simulink model "FOC_Test"  (R2022b)
settings: Solver=FixedStepDiscrete  StartTime=0.0  StopTime=10.0  FixedStep=0.0001  RelTol=1e-3
libraries: Rtunit12 x30, PowerElectronics x2, simulink x1, RtuBox x1
settings Model: Creator=LJ  LastModifiedBy=Administrator
settings SolverCC: AlgebraicLoopSolver=TrustRegion
settings DataIOCC: ReturnWorkspaceOutputs=off
settings OptimizationCC: ReuseModelBlockBuffer=on
settings DebuggingCC: UnderspecifiedInitializationDetection=Classic  MergeDetectMultiDrivingBlocksExec=none  UnconnectedInputMsg=warning  UnconnectedOutputMsg=warning  UnconnectedLineMsg=warning  ArithmeticOperatorsInVariantConditions=warning
settings ModelReferenceCC: EnableRefExpFcnMdlSchedulingChecks=on
settings SFSimCC: SimUseLocalCustomCode=off  CustomCodeUndefinedFunction=UseInterfaceOnly
settings RTWCC: RTWUseLocalCustomCode=off
settings CodeAppCC: StateflowObjectComments=on

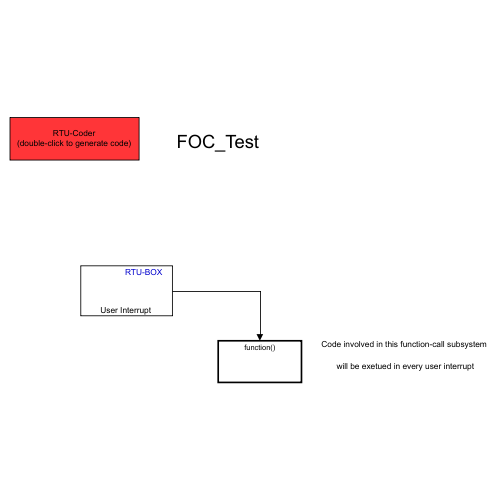
[thumbnail: Simulink's stored preview of the top-level diagram]
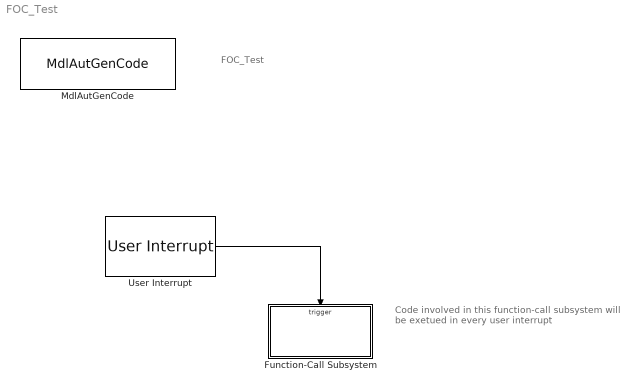
== system FOC_Test ==
  note: Code involved in this function-call subsystem
      |
      | will be exetued in every user interrupt
  note: FOC_Test
  Function-Call Subsystem : Subsystem  TreatAsAtomicUnit=on
  MdlAutGenCode : RtuBox/MdlAutGenCode
      settings: SourceProductName=RTU-BOX204 Toolbox
  User Interrupt : Rtunit12/User Interrupt  TimeEnable=User setting  TimeFreq=10
      settings: SourceProductName=RTU-BOX204 Toolbox
  wires:
  User Interrupt/1 -> Function-Call Subsystem/Trigger

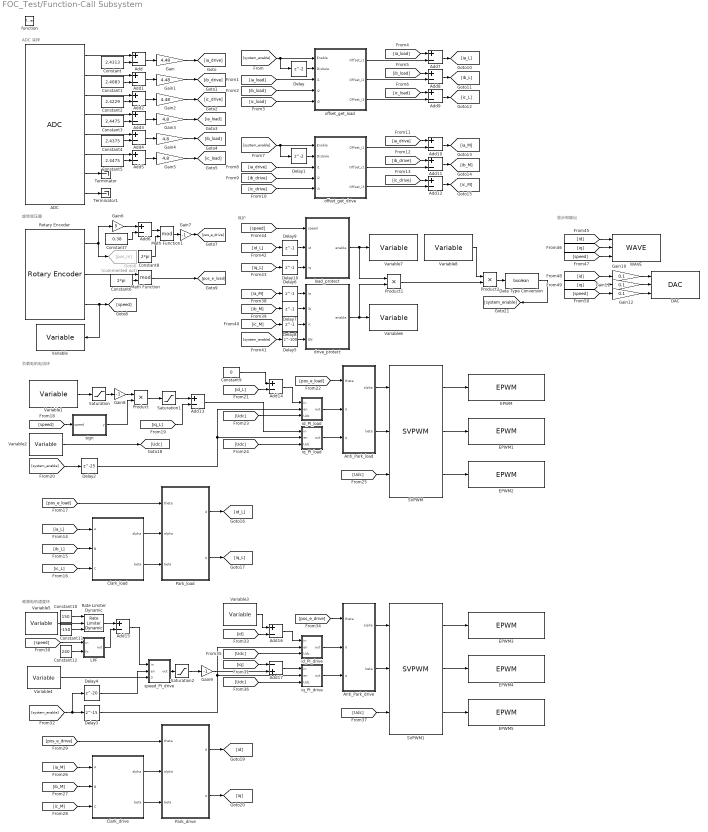
== system FOC_Test/Function-Call Subsystem ==
  note: 显示和输出
  note: 保护
  note: 负载电机电流环
  note: 旋转变压器
  note: ADC 采样
  note: 被测电机速度环
  function : TriggerPort  TriggerType=function-call  VariantControl=Variant
  " SVPWM" : PowerElectronics/ SVPWM
      settings: SourceProductName=RTU-BOX204 Toolbox
  " SVPWM1" : PowerElectronics/ SVPWM
      settings: SourceProductName=RTU-BOX204 Toolbox
  ADC : Rtunit12/ADC  SlotNo=ADC_A  InputSingleType=Single ended input and 16-bit resolution  numConversionsSingle=8  conv0=ADCIN00  GainEable1=on  Gain1=0.00030517578125  Offset1=0  conv1=ADCIN01  GainEable2=on  Gain2=0.00030517578125  Offset2=0  conv2=ADCIN02  GainEable3=on  Gain3=0.00030517578125  Offset3=0  conv3=ADCIN03  GainEable4=on  Gain4=0.00030517578125  Offset4=0  conv4=ADCIN04  GainEable5=on  Gain5=0.00030517578125  Offset5=0  conv5=ADCIN05  GainEable6=on  Gain6=0.00030517578125  Offset6=0  conv6=ADCIN06  GainEable7=on  Gain7=0.00030517578125  Offset7=0  conv7=ADCIN07  GainEable8=on  Gain8=0.00030517578125  Offset8=0  conv8=ADCIN01  GainEable9=off  Gain9=0.00015411376953125  Offset9=0  conv9=ADCIN01  GainEable10=off  Gain10=0.00015411376953125  Offset10=0  conv10=ADCIN01  GainEable11=off  Gain11=0.00015411376953125  Offset11=0  conv11=ADCIN01  GainEable12=off  Gain12=0.00015411376953125  Offset12=0  conv12=ADCIN01  GainEable13=off  Gain13=0.00015411376953125  Offset13=0  conv13=ADCIN01  GainEable14=off  Gain14=0.00015411376953125  Offset14=0  conv14=ADCIN01  GainEable15=off  Gain15=0.00015411376953125  Offset15=0  conv15=ADCIN01  GainEable16=off  Gain16=0.00015411376953125  Offset16=0  c28xmultiPort=on  AutoOffset=off
      settings: SourceProductName=RTU-BOX204 Toolbox
  Add{,1..16} (17 alike) : Sum  Inputs=+-  OutDataTypeStr=single  AccumDataTypeStr=single
  Add17 : Sum  Inputs=-+  OutDataTypeStr=single  AccumDataTypeStr=single
  Anti_Park_drive : MATLAB Function  TreatAsAtomicUnit=on
  Anti_Park_load : MATLAB Function  TreatAsAtomicUnit=on
  Clark_drive : MATLAB Function  TreatAsAtomicUnit=on
  Clark_load : MATLAB Function  TreatAsAtomicUnit=on
  Constant : Constant  Value=2.4313  OutDataTypeStr=single
  Constant1 : Constant  Value=2.4083  OutDataTypeStr=single
  Constant10 : Constant  Value=150  OutDataTypeStr=single
  Constant11 : Constant  Value=-150  OutDataTypeStr=single
  Constant12 : Constant  Value=240  OutDataTypeStr=single
  Constant2 : Constant  Value=2.4229  OutDataTypeStr=single
  Constant3 : Constant  Value=2.4475  OutDataTypeStr=single
  Constant4 : Constant  Value=2.4375  OutDataTypeStr=single
  Constant5 : Constant  Value=2.4475  OutDataTypeStr=single
  Constant6 : Constant  Value=2*pi  OutDataTypeStr=single
  Constant7 : Constant  Value=0.38  OutDataTypeStr=single
  Constant8 : Constant  Value=2*pi  OutDataTypeStr=single
  Constant9 : Constant  Value=0  OutDataTypeStr=single
  DAC : Rtunit12/DAC  useModule=A  Ts=-1  numConversionsSingle=3  conv0=DACOUTA0  conv1=DACOUTA1  conv2=DACOUTA2  conv3=DACOUTA0  conv4=DACOUTA0  conv5=DACOUTA0  conv6=DACOUTA0  conv7=DACOUTA0  conv8=DACOUT00  conv9=DACOUT00  conv10=DACOUT00  conv11=DACOUT00  conv12=DACOUT00  conv13=DACOUT00  conv14=DACOUT00  conv15=DACOUT00  dType=uint32  c28xmultiPort=on
      settings: SourceProductName=RTU-BOX204 Toolbox
  Data Type Conversion : DataTypeConversion  OutDataTypeStr=boolean  SaturateOnIntegerOverflow=off  RndMeth=Floor
  Delay : Delay  InitialCondition=0
  Delay1 : Delay  InitialCondition=0
  Delay{6..10} (5 alike) : Delay  DelayLength=1  InitialCondition=0
  Delay2 : Delay  DelayLength=25  InitialCondition=0
  Delay3 : Delay  DelayLength=15  InitialCondition=0
  Delay4 : Delay  DelayLength=20  InitialCondition=0
  Delay5 : Delay  DelayLength=100  InitialCondition=0
  EPWM : Rtunit12/EPWM  UserMode=Complimentary Signals Output  CHANNEL=4  EPWMA=EPWMA  LoadmodeA=CNT=0  LoadmodeB=CNT=0  STYLE=Triangle  DEADTIME=1  PhaseEnable=OFF  PhaseSlct=Dialog  PHASE=0  FreqSlct=Dialog  Frequency=10000  DutyUnit=Percentages  DutyInit=0.5  SynEnable=CTR=Zero  ChoppEnable=OFF  ChoppFrqDivd=5  ChoppCycFir=1  ChoppPulseCyc=1
      settings: SourceProductName=RTU-BOX204 Toolbox
  EPWM1 : Rtunit12/EPWM  UserMode=Complimentary Signals Output  CHANNEL=5  EPWMA=EPWMA  LoadmodeA=CNT=0  LoadmodeB=CNT=0  STYLE=Triangle  DEADTIME=1  PhaseEnable=ON  PhaseSlct=Dialog  PHASE=0  FreqSlct=Dialog  Frequency=10000  DutyUnit=Percentages  DutyInit=0.5  SynEnable=Synchronization Input  ChoppEnable=OFF  ChoppFrqDivd=5  ChoppCycFir=1  ChoppPulseCyc=1
      settings: SourceProductName=RTU-BOX204 Toolbox
  EPWM2 : Rtunit12/EPWM  UserMode=Complimentary Signals Output  CHANNEL=6  EPWMA=EPWMA  LoadmodeA=CNT=0  LoadmodeB=CNT=0  STYLE=Triangle  DEADTIME=1  PhaseEnable=ON  PhaseSlct=Dialog  PHASE=0  FreqSlct=Dialog  Frequency=10000  DutyUnit=Percentages  DutyInit=0.5  SynEnable=Synchronization Input  ChoppEnable=OFF  ChoppFrqDivd=5  ChoppCycFir=1  ChoppPulseCyc=1
      settings: SourceProductName=RTU-BOX204 Toolbox
  EPWM3 : Rtunit12/EPWM  UserMode=Complimentary Signals Output  CHANNEL=1  EPWMA=EPWMA  LoadmodeA=CNT=0  LoadmodeB=CNT=0  STYLE=Triangle  DEADTIME=1  PhaseEnable=OFF  PhaseSlct=Dialog  PHASE=0  FreqSlct=Dialog  Frequency=10000  DutyUnit=Percentages  DutyInit=0.5  SynEnable=CTR=Zero  ChoppEnable=OFF  ChoppFrqDivd=5  ChoppCycFir=1  ChoppPulseCyc=1
      settings: SourceProductName=RTU-BOX204 Toolbox
  EPWM4 : Rtunit12/EPWM  UserMode=Complimentary Signals Output  CHANNEL=2  EPWMA=EPWMA  LoadmodeA=CNT=0  LoadmodeB=CNT=0  STYLE=Triangle  DEADTIME=1  PhaseEnable=ON  PhaseSlct=Dialog  PHASE=0  FreqSlct=Dialog  Frequency=10000  DutyUnit=Percentages  DutyInit=0.5  SynEnable=Synchronization Input  ChoppEnable=OFF  ChoppFrqDivd=5  ChoppCycFir=1  ChoppPulseCyc=1
      settings: SourceProductName=RTU-BOX204 Toolbox
  EPWM5 : Rtunit12/EPWM  UserMode=Complimentary Signals Output  CHANNEL=3  EPWMA=EPWMA  LoadmodeA=CNT=0  LoadmodeB=CNT=0  STYLE=Triangle  DEADTIME=1  PhaseEnable=ON  PhaseSlct=Dialog  PHASE=0  FreqSlct=Dialog  Frequency=10000  DutyUnit=Percentages  DutyInit=0.5  SynEnable=Synchronization Input  ChoppEnable=OFF  ChoppFrqDivd=5  ChoppCycFir=1  ChoppPulseCyc=1
      settings: SourceProductName=RTU-BOX204 Toolbox
  Gain : Gain  Gain=4.48  ParamDataTypeStr=single  OutDataTypeStr=single
  Gain1 : Gain  Gain=4.48  ParamDataTypeStr=single  OutDataTypeStr=single
  Gain10 : Gain  Gain=0.1  ParamDataTypeStr=single  OutDataTypeStr=single
  Gain11 : Gain  Gain=0.1  ParamDataTypeStr=single  OutDataTypeStr=single
  Gain12 : Gain  Gain=0.1  ParamDataTypeStr=single  OutDataTypeStr=single
  Gain2 : Gain  Gain=4.48  ParamDataTypeStr=single  OutDataTypeStr=single
  Gain3 : Gain  Gain=4.8  ParamDataTypeStr=single  OutDataTypeStr=single
  Gain4 : Gain  Gain=4.8  ParamDataTypeStr=single  OutDataTypeStr=single
  Gain5 : Gain  Gain=4.8  ParamDataTypeStr=single  OutDataTypeStr=single
  Gain6 : Gain  Gain=5  ParamDataTypeStr=single  OutDataTypeStr=single
  Gain7 : Gain  Gain=-1  ParamDataTypeStr=single  OutDataTypeStr=single
  Gain8 : Gain  Gain=-1  ParamDataTypeStr=single  OutDataTypeStr=single
  Gain9 : Gain  Gain=-1  ParamDataTypeStr=single  OutDataTypeStr=single
  Goto6 : Goto  Commented=on  GotoTag=pos_m
  LPF : Subsystem
  Math Function : Math  Operator=mod
  Math Function1 : Math  Operator=mod
  Park_drive : MATLAB Function  TreatAsAtomicUnit=on
  Park_load : MATLAB Function  TreatAsAtomicUnit=on
  Product : Product  OutDataTypeStr=single
  Product1 : Product  OutDataTypeStr=single
  Product2 : Product  OutDataTypeStr=single
  Rate Limiter Dynamic : simulink/Discontinuities/Rate Limiter Dynamic
  Rotary Encoder : Rtunit12/Rotary Encoder  ChipSlct=0  Position_Compensate=0  Pole=4  Pole_Encoder=1  Bit_Encoder=16
      settings: SourceProductName=RTU-BOX204 Toolbox
  Saturation : Saturate  UpperLimit=1  LowerLimit=-1  OutDataTypeStr=single
  Saturation1 : Saturate  UpperLimit=2  LowerLimit=-2  OutDataTypeStr=single
  Saturation2 : Saturate  UpperLimit=3  LowerLimit=-3  OutDataTypeStr=single
  Terminator : Terminator
  Terminator1 : Terminator
  Variable : Rtunit12/Variable  nameStr=speed  DType=Single  Rw=Read only  InitVale=2  uint=rpm
      settings: SourceProductName=RTU-BOX204 Toolbox
  Variable1 : Rtunit12/Variable  nameStr=iq_load_ref  DType=Single  Rw=Read and Write  InitVale=0  uint=A
      settings: SourceProductName=RTU-BOX204 Toolbox
  Variable2 : Rtunit12/Variable  nameStr=Udc  DType=Single  Rw=Read and Write  InitVale=60  uint=V
      settings: SourceProductName=RTU-BOX204 Toolbox
  Variable3 : Rtunit12/Variable  nameStr=id_ref  DType=Single  Rw=Read and Write  InitVale=0  uint=A
      settings: SourceProductName=RTU-BOX204 Toolbox
  Variable4 : Rtunit12/Variable  nameStr=iq_limit  DType=Single  Rw=Read and Write  InitVale=3  uint=A
      settings: SourceProductName=RTU-BOX204 Toolbox
  Variable5 : Rtunit12/Variable  nameStr=speed_ref  DType=Single  Rw=Read and Write  InitVale=0  uint=rpm
      settings: SourceProductName=RTU-BOX204 Toolbox
  Variable6 : Rtunit12/Variable  nameStr=drive_motor_protect  DType=Single  Rw=Read only  InitVale=2
      settings: SourceProductName=RTU-BOX204 Toolbox
  Variable7 : Rtunit12/Variable  nameStr=load_motor_protect  DType=Single  Rw=Read only  InitVale=2
      settings: SourceProductName=RTU-BOX204 Toolbox
  Variable8 : Rtunit12/Variable  nameStr=system_enable  DType=Boolean  Rw=Read and Write  InitVale=0
      settings: SourceProductName=RTU-BOX204 Toolbox
  WAVE : Rtunit12/WAVE  RcvMode=Rtunit Studio  NumChnnl=3  Wave1Name=id  Wave1Max=4  Wave1Min=-4  Wave2Name=iq  Wave2Max=4  Wave2Min=-4  Wave3Name=speed  Wave3Max=600  Wave3Min=-600  Wave4Name=wave4  Wave4Max=10  Wave4Min=-10  Wave5Name=wave5  Wave5Max=10  Wave5Min=-10  Wave6Name=wave6  Wave6Max=10  Wave6Min=-10  Wave7Name=wave7  Wave7Max=10  Wave7Min=-10  Wave8Name=wave8  Wave8Max=10  Wave8Min=-10
      settings: SourceProductName=RTU-BOX204 Toolbox
  drive_protect : MATLAB Function  TreatAsAtomicUnit=on
  id_PI_drive : Subsystem
  id_PI_load : Subsystem
  iq_PI_drive : Subsystem
  iq_PI_load : Subsystem
  load_protect : MATLAB Function  TreatAsAtomicUnit=on
  offset_get_drive : MATLAB Function  TreatAsAtomicUnit=on
  offset_get_load : MATLAB Function  TreatAsAtomicUnit=on
  sign : MATLAB Function  TreatAsAtomicUnit=on
  speed_PI_drive : Subsystem
  wires:
  Constant/1 -> Add/2
  ADC/1 -> Add/1
  Add/1 -> Gain/1
  Gain/1 -> [ia_drive]
  Constant1/1 -> Add1/2
  Gain1/1 -> [ib_drive]
  ADC/2 -> Add1/1
  Add1/1 -> Gain1/1
  Add2/1 -> Gain2/1
  ADC/3 -> Add2/1
  Constant2/1 -> Add2/2
  Gain2/1 -> [ic_drive]
  Gain5/1 -> [ic_load]
  Constant5/1 -> Add5/2
  Constant3/1 -> Add3/2
  Add5/1 -> Gain5/1
  Gain3/1 -> [ia_load]
  Add4/1 -> Gain4/1
  ADC/5 -> Add4/1
  Constant4/1 -> Add4/2
  Gain4/1 -> [ib_load]
  ADC/6 -> Add5/1
  ADC/4 -> Add3/1
  Add3/1 -> Gain3/1
  ADC/7 -> Terminator/1
  ADC/8 -> Terminator1/1
  Rotary Encoder/1 -> Gain6/1, Goto6/1
  Rotary Encoder/2 -> Math Function/1
  Rotary Encoder/3 -> Variable/1, [speed]
  Constant6/1 -> Math Function/2
  Math Function/1 -> [pos_e_load]
  Gain6/1 -> Add6/1
  Constant7/1 -> Add6/2
  Add6/1 -> Math Function1/1
  Math Function1/1 -> Gain7/1
  Constant8/1 -> Math Function1/2
  Gain7/1 -> [pos_e_drive]
  [system_enable] -> Delay/1, offset_get_load/1(Enable)
  Delay/1 -> offset_get_load/2(Disbale)
  [ia_load] -> offset_get_load/3(i1)
  [ic_load] -> offset_get_load/5(i3)
  [ib_load] -> offset_get_load/4(i2)
  offset_get_load/1(Offset_i1) -> Add7/2
  [ia_load] -> Add7/1
  offset_get_load/2(Offset_i2) -> Add8/2
  [ib_load] -> Add8/1
  [ic_load] -> Add9/1
  offset_get_load/3(Offset_i3) -> Add9/2
  Add7/1 -> [ia_L]
  Add8/1 -> [ib_L]
  Add9/1 -> [ic_L]
  offset_get_drive/1(Offset_i1) -> Add10/2
  offset_get_drive/3(Offset_i3) -> Add12/2
  [ib_drive] -> Add11/1
  Add10/1 -> [ia_M]
  offset_get_drive/2(Offset_i2) -> Add11/2
  [ia_drive] -> Add10/1
  Add12/1 -> [ic_M]
  [system_enable] -> Delay1/1, offset_get_drive/1(Enable)
  [ic_drive] -> offset_get_drive/5(i3)
  Add11/1 -> [ib_M]
  [ia_drive] -> offset_get_drive/3(i1)
  Delay1/1 -> offset_get_drive/2(Disbale)
  [ib_drive] -> offset_get_drive/4(i2)
  [ic_drive] -> Add12/1
  [ia_L] -> Clark_load/1(A)
  [ib_L] -> Clark_load/2(B)
  [ic_L] -> Clark_load/3(C)
  Clark_load/1(alpha) -> Park_load/2(alpha)
  Clark_load/2(beta) -> Park_load/3(beta)
  [pos_e_load] -> Park_load/1(theta)
  Park_load/1(d) -> [id_L]
  Park_load/2(q) -> [iq_L]
  Variable1/1 -> Saturation/1
  Saturation/1 -> Gain8/1
  Gain8/1 -> Product/1
  sign/1(y) -> Product/2
  [speed] -> sign/1(speed)
  Product/1 -> Saturation1/1
  Saturation1/1 -> Add13/1
  [iq_L] -> Add13/2
  [system_enable] -> Delay2/1
  Delay2/1 -> id_PI_load/2(en), iq_PI_load/2(en)
  Add13/1 -> iq_PI_load/1(in)
  [id_L] -> Add14/2
  Add14/1 -> id_PI_load/1(in)
  Constant9/1 -> Add14/1
  id_PI_load/1(out) -> Anti_Park_load/2(d)
  iq_PI_load/1(out) -> Anti_Park_load/3(q)
  [pos_e_load] -> Anti_Park_load/1(theta)
  Variable2/1 -> [Udc]
  [Udc] -> id_PI_load/3(Udc)
  [Udc] -> iq_PI_load/3(Udc)
  Anti_Park_load/1(alpha) -> " SVPWM"/1
  Anti_Park_load/2(beta) -> " SVPWM"/2
  [Udc] -> " SVPWM"/3
  " SVPWM"/1 -> EPWM/1
  " SVPWM"/2 -> EPWM1/1
  " SVPWM"/3 -> EPWM2/1
  " SVPWM1"/2 -> EPWM4/1
  " SVPWM1"/3 -> EPWM5/1
  [id] -> Add16/2
  [pos_e_drive] -> Anti_Park_drive/1(theta)
  iq_PI_drive/1(out) -> Anti_Park_drive/3(q)
  Anti_Park_drive/1(alpha) -> " SVPWM1"/1
  [Udc] -> id_PI_drive/3(Udc)
  [Udc] -> " SVPWM1"/3
  Variable3/1 -> Add16/1
  Delay3/1 -> id_PI_drive/2(en), iq_PI_drive/2(en)
  Anti_Park_drive/2(beta) -> " SVPWM1"/2
  [Udc] -> iq_PI_drive/3(Udc)
  [pos_e_drive] -> Park_drive/1(theta)
  id_PI_drive/1(out) -> Anti_Park_drive/2(d)
  Clark_drive/1(alpha) -> Park_drive/2(alpha)
  Park_drive/1(d) -> [id]
  Park_drive/2(q) -> [iq]
  Clark_drive/2(beta) -> Park_drive/3(beta)
  [ic_M] -> Clark_drive/3(C)
  Add16/1 -> id_PI_drive/1(in)
  " SVPWM1"/1 -> EPWM3/1
  [system_enable] -> Delay4/1, Delay3/1
  [ib_M] -> Clark_drive/2(B)
  [ia_M] -> Clark_drive/1(A)
  Saturation2/1 -> Gain9/1
  speed_PI_drive/1(out) -> Saturation2/1
  Delay4/1 -> speed_PI_drive/2(en)
  Variable4/1 -> speed_PI_drive/3(iq_limit)
  Rate Limiter Dynamic/1 -> Add15/1
  Add15/1 -> speed_PI_drive/1(in)
  Variable5/1 -> Rate Limiter Dynamic/2
  Constant10/1 -> Rate Limiter Dynamic/1
  Constant11/1 -> Rate Limiter Dynamic/3
  LPF/1(out) -> Add15/2
  Constant12/1 -> LPF/2(fc)
  [speed] -> LPF/1(in)
  Gain9/1 -> Add17/2
  Add17/1 -> iq_PI_drive/1(in)
  [iq] -> Add17/1
  [system_enable] -> Delay5/1
  Delay5/1 -> drive_protect/4(EN)
  [ia_M] -> Delay6/1
  Delay6/1 -> drive_protect/1(ia)
  [ib_M] -> Delay7/1
  Delay7/1 -> drive_protect/2(ib)
  [ic_M] -> Delay8/1
  Delay8/1 -> drive_protect/3(ic)
  drive_protect/1(enable) -> Product1/2, Variable6/1
  [speed] -> load_protect/1(speed)
  load_protect/1(enable) -> Product1/1, Variable7/1
  Product1/1 -> Product2/2
  Variable8/1 -> Product2/1
  [speed] -> WAVE/3
  [iq] -> WAVE/2
  [id] -> WAVE/1
  [id] -> Gain10/1
  Gain10/1 -> DAC/1
  [iq] -> Gain11/1
  Gain11/1 -> DAC/2
  [speed] -> Gain12/1
  Gain12/1 -> DAC/3
  Product2/1 -> Data Type Conversion/1
  Data Type Conversion/1 -> [system_enable]
  [id_L] -> Delay9/1
  Delay9/1 -> load_protect/2(id)
  [iq_L] -> Delay10/1
  Delay10/1 -> load_protect/3(iq)

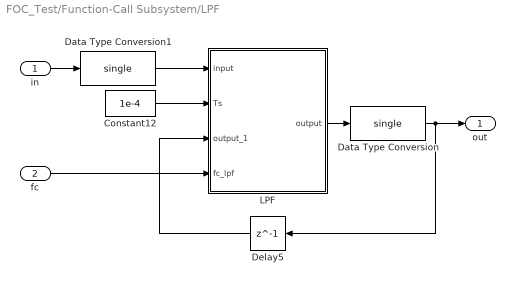
== system FOC_Test/Function-Call Subsystem/LPF ==
  in : Inport
  fc : Inport  Port=2
  Constant12 : Constant  Value=1e-4  OutDataTypeStr=single
  Data Type Conversion : DataTypeConversion  OutDataTypeStr=single  SaturateOnIntegerOverflow=off  RndMeth=Floor
  Data Type Conversion1 : DataTypeConversion  OutDataTypeStr=single  SaturateOnIntegerOverflow=off  RndMeth=Floor
  Delay5 : Delay  DelayLength=1  InitialCondition=0
  LPF : MATLAB Function  TreatAsAtomicUnit=on
  out : Outport
  wires:
  Data Type Conversion/1 -> out/1, Delay5/1
  in/1 -> Data Type Conversion1/1
  Delay5/1 -> LPF/3(output_1)
  Data Type Conversion1/1 -> LPF/1(input)
  fc/1 -> LPF/4(fc_lpf)
  Constant12/1 -> LPF/2(Ts)
  LPF/1(output) -> Data Type Conversion/1

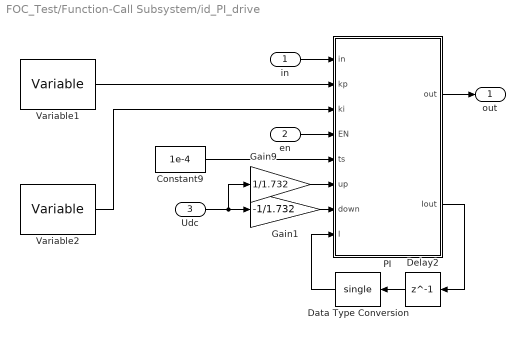
== system FOC_Test/Function-Call Subsystem/id_PI_drive ==
  in : Inport
  en : Inport  Port=2
  Udc : Inport  Port=3
  Constant9 : Constant  Value=1e-4  OutDataTypeStr=single
  Data Type Conversion : DataTypeConversion  OutDataTypeStr=single  SaturateOnIntegerOverflow=off  RndMeth=Floor
  Delay2 : Delay  DelayLength=1  InitialCondition=0
  Gain1 : Gain  Gain=-1/1.732  ParamDataTypeStr=single  OutDataTypeStr=single
  Gain9 : Gain  Gain=1/1.732  ParamDataTypeStr=single  OutDataTypeStr=single
  PI : MATLAB Function  TreatAsAtomicUnit=on
  Variable1 : Rtunit12/Variable  nameStr=id_Kp_drive  DType=Single  Rw=Read and Write  InitVale=20
      settings: SourceProductName=RTU-BOX204 Toolbox
  Variable2 : Rtunit12/Variable  nameStr=id_Ki_drive  DType=Single  Rw=Read and Write  InitVale=3000
      settings: SourceProductName=RTU-BOX204 Toolbox
  out : Outport
  wires:
  Delay2/1 -> Data Type Conversion/1
  Data Type Conversion/1 -> PI/8(I)
  Udc/1 -> Gain1/1, Gain9/1
  Variable1/1 -> PI/2(kp)
  PI/2(Iout) -> Delay2/1
  en/1 -> PI/4(EN)
  in/1 -> PI/1(in)
  Variable2/1 -> PI/3(ki)
  Constant9/1 -> PI/5(ts)
  PI/1(out) -> out/1
  Gain1/1 -> PI/7(down)
  Gain9/1 -> PI/6(up)

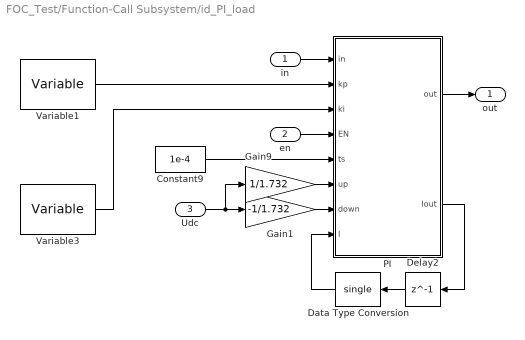
== system FOC_Test/Function-Call Subsystem/id_PI_load ==
  in : Inport
  en : Inport  Port=2
  Udc : Inport  Port=3
  Constant9 : Constant  Value=1e-4  OutDataTypeStr=single
  Data Type Conversion : DataTypeConversion  OutDataTypeStr=single  SaturateOnIntegerOverflow=off  RndMeth=Floor
  Delay2 : Delay  DelayLength=1  InitialCondition=0
  Gain1 : Gain  Gain=-1/1.732  ParamDataTypeStr=single  OutDataTypeStr=single
  Gain9 : Gain  Gain=1/1.732  ParamDataTypeStr=single  OutDataTypeStr=single
  PI : MATLAB Function  TreatAsAtomicUnit=on
  Variable1 : Rtunit12/Variable  nameStr=id_Kp_load  DType=Single  Rw=Read and Write  InitVale=10
      settings: SourceProductName=RTU-BOX204 Toolbox
  Variable3 : Rtunit12/Variable  nameStr=id_Ki_load  DType=Single  Rw=Read and Write  InitVale=150
      settings: SourceProductName=RTU-BOX204 Toolbox
  out : Outport
  wires:
  Delay2/1 -> Data Type Conversion/1
  Data Type Conversion/1 -> PI/8(I)
  Variable1/1 -> PI/2(kp)
  PI/2(Iout) -> Delay2/1
  en/1 -> PI/4(EN)
  in/1 -> PI/1(in)
  Variable3/1 -> PI/3(ki)
  Constant9/1 -> PI/5(ts)
  PI/1(out) -> out/1
  Gain9/1 -> PI/6(up)
  Gain1/1 -> PI/7(down)
  Udc/1 -> Gain1/1, Gain9/1

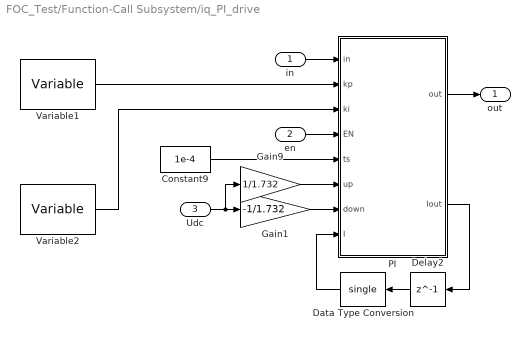
== system FOC_Test/Function-Call Subsystem/iq_PI_drive ==
  in : Inport
  en : Inport  Port=2
  Udc : Inport  Port=3
  Constant9 : Constant  Value=1e-4  OutDataTypeStr=single
  Data Type Conversion : DataTypeConversion  OutDataTypeStr=single  SaturateOnIntegerOverflow=off  RndMeth=Floor
  Delay2 : Delay  DelayLength=1  InitialCondition=0
  Gain1 : Gain  Gain=-1/1.732  ParamDataTypeStr=single  OutDataTypeStr=single
  Gain9 : Gain  Gain=1/1.732  ParamDataTypeStr=single  OutDataTypeStr=single
  PI : MATLAB Function  TreatAsAtomicUnit=on
  Variable1 : Rtunit12/Variable  nameStr=iq_Kp_drive  DType=Single  Rw=Read and Write  InitVale=20
      settings: SourceProductName=RTU-BOX204 Toolbox
  Variable2 : Rtunit12/Variable  nameStr=iq_Ki_drive  DType=Single  Rw=Read and Write  InitVale=3000
      settings: SourceProductName=RTU-BOX204 Toolbox
  out : Outport
  wires:
  Delay2/1 -> Data Type Conversion/1
  Data Type Conversion/1 -> PI/8(I)
  Gain9/1 -> PI/6(up)
  Udc/1 -> Gain9/1, Gain1/1
  Variable1/1 -> PI/2(kp)
  PI/2(Iout) -> Delay2/1
  en/1 -> PI/4(EN)
  in/1 -> PI/1(in)
  Variable2/1 -> PI/3(ki)
  Constant9/1 -> PI/5(ts)
  PI/1(out) -> out/1
  Gain1/1 -> PI/7(down)

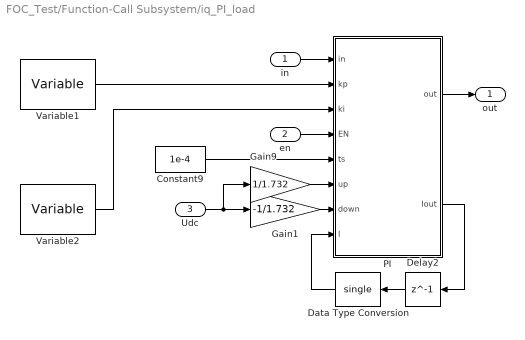
== system FOC_Test/Function-Call Subsystem/iq_PI_load ==
  in : Inport
  en : Inport  Port=2
  Udc : Inport  Port=3
  Constant9 : Constant  Value=1e-4  OutDataTypeStr=single
  Data Type Conversion : DataTypeConversion  OutDataTypeStr=single  SaturateOnIntegerOverflow=off  RndMeth=Floor
  Delay2 : Delay  DelayLength=1  InitialCondition=0
  Gain1 : Gain  Gain=-1/1.732  ParamDataTypeStr=single  OutDataTypeStr=single
  Gain9 : Gain  Gain=1/1.732  ParamDataTypeStr=single  OutDataTypeStr=single
  PI : MATLAB Function  TreatAsAtomicUnit=on
  Variable1 : Rtunit12/Variable  nameStr=iq_Kp_load  DType=Single  Rw=Read and Write  InitVale=10
      settings: SourceProductName=RTU-BOX204 Toolbox
  Variable2 : Rtunit12/Variable  nameStr=iq_Ki_load  DType=Single  Rw=Read and Write  InitVale=150
      settings: SourceProductName=RTU-BOX204 Toolbox
  out : Outport
  wires:
  Delay2/1 -> Data Type Conversion/1
  Data Type Conversion/1 -> PI/8(I)
  Gain9/1 -> PI/6(up)
  Udc/1 -> Gain9/1, Gain1/1
  Variable1/1 -> PI/2(kp)
  PI/2(Iout) -> Delay2/1
  en/1 -> PI/4(EN)
  in/1 -> PI/1(in)
  Variable2/1 -> PI/3(ki)
  Constant9/1 -> PI/5(ts)
  PI/1(out) -> out/1
  Gain1/1 -> PI/7(down)

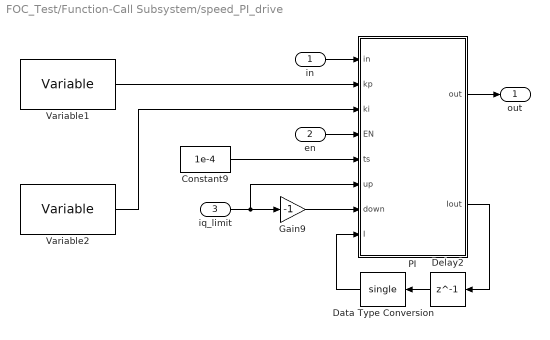
== system FOC_Test/Function-Call Subsystem/speed_PI_drive ==
  in : Inport
  en : Inport  Port=2
  iq_limit : Inport  Port=3
  Constant9 : Constant  Value=1e-4  OutDataTypeStr=single
  Data Type Conversion : DataTypeConversion  OutDataTypeStr=single  SaturateOnIntegerOverflow=off  RndMeth=Floor
  Delay2 : Delay  DelayLength=1  InitialCondition=0
  Gain9 : Gain  Gain=-1  ParamDataTypeStr=single  OutDataTypeStr=single
  PI : MATLAB Function  TreatAsAtomicUnit=on
  Variable1 : Rtunit12/Variable  nameStr=speed_Kp_drive  DType=Single  Rw=Read and Write  InitVale=0.005
      settings: SourceProductName=RTU-BOX204 Toolbox
  Variable2 : Rtunit12/Variable  nameStr=speed_Ki_drive  DType=Single  Rw=Read and Write  InitVale=0.05
      settings: SourceProductName=RTU-BOX204 Toolbox
  out : Outport
  wires:
  Delay2/1 -> Data Type Conversion/1
  Data Type Conversion/1 -> PI/8(I)
  Variable1/1 -> PI/2(kp)
  PI/2(Iout) -> Delay2/1
  en/1 -> PI/4(EN)
  in/1 -> PI/1(in)
  Variable2/1 -> PI/3(ki)
  Constant9/1 -> PI/5(ts)
  PI/1(out) -> out/1
  Gain9/1 -> PI/7(down)
  iq_limit/1 -> PI/6(up), Gain9/1

== matlab function FOC_Test/Function-Call Subsystem/Anti_Park_load ==
  data: theta input; alpha output; d input; q input; beta output
function [alpha, beta] = Anti_Park(theta, d, q)

alpha = cos(theta) * d - sin(theta) * q;
beta = sin(theta) * d + cos(theta) * q;

end

== matlab function FOC_Test/Function-Call Subsystem/Anti_Park_drive ==
  data: theta input; alpha output; d input; q input; beta output
function [alpha, beta] =Anti_Park(theta, d, q)

alpha = cos(theta) * d - sin(theta) * q;
beta = sin(theta) * d + cos(theta) * q;

end

== matlab function FOC_Test/Function-Call Subsystem/Clark_drive ==
  data: A input; alpha output; B input; C input; beta output
function [alpha, beta] = Clark(A, B, C)

alpha = 2/3 * (A - 0.5 * (B + C));
beta = 2/3 * (sqrt(3)/2 * (B - C));

end

== matlab function FOC_Test/Function-Call Subsystem/Park_drive ==
  data: theta input; d output; alpha input; beta input; q output
function [d, q] = Park(theta, alpha, beta)

d = cos(theta) * alpha + sin(theta) * beta;
q = -sin(theta) * alpha + cos(theta) * beta;

end

== matlab function FOC_Test/Function-Call Subsystem/id_PI_drive/PI ==
  data: in input; out output; kp input; ki input; Iout output; EN input; ts input; up input; down input; I input
function [out, Iout] = PI(in, kp, ki, EN, ts, up, down, I)

if(EN == 1)

    % 计算积分输出
    Iout = I + ki * ts * in;

    % 积分限幅
    if(Iout > up)
        Iout = up;
    end
    if(Iout < down)
        Iout = down;
    end
    
    % 合并积分输出和比例输出
    out = kp * in + Iout; 

    % 输出限幅
    if(out > up)
        out = up;
    end
    if(out < down)
        out = down;
    end
else
    Iout = single(0);
    out = single(0);
end
end

== matlab function FOC_Test/Function-Call Subsystem/iq_PI_drive/PI ==
  data: in input; out output; kp input; ki input; Iout output; EN input; ts input; up input; down input; I input
function [out, Iout] = PI(in, kp, ki, EN, ts, up, down, I)

if(EN == 1)

    % 计算积分输出
    Iout = I + ki * ts * in;

    % 积分限幅
    if(Iout > up)
        Iout = up;
    end
    if(Iout < down)
        Iout = down;
    end
    
    % 合并积分输出和比例输出
    out = kp * in + Iout; 

    % 输出限幅
    if(out > up)
        out = up;
    end
    if(out < down)
        out = down;
    end
else
    Iout = single(0);
    out = single(0);
end
end

== matlab function FOC_Test/Function-Call Subsystem/speed_PI_drive/PI ==
  data: in input; out output; kp input; ki input; Iout output; EN input; ts input; up input; down input; I input
function [out, Iout] = PI(in, kp, ki, EN, ts, up, down, I)

if(EN == 1)

    % 计算积分输出
    Iout = I + ki * ts * in;

    % 积分限幅
    if(Iout > up)
        Iout = up;
    end
    if(Iout < down)
        Iout = down;
    end
    
    % 合并积分输出和比例输出
    out = kp * in + Iout; 

    % 输出限幅
    if(out > up)
        out = up;
    end
    if(out < down)
        out = down;
    end
else
    Iout = single(0);
    out = single(0);
end
end

== matlab function FOC_Test/Function-Call Subsystem/offset_get_drive ==
  data: Enable input; Offset_i1 output; Disbale input; i1 input; i2 input; i3 input; Offset_i2 output; Offset_i3 output
% 使能时采集电流偏置(采集最近的一次)
function [Offset_i1, Offset_i2, Offset_i3]= offset_get(Enable, Disbale, i1, i2, i3)

% ia1, ib1, ic1 是锁存变量
persistent ia1 ib1 ic1

% 初始化
if isempty(ia1)
    ia1 = single(0);
end
if isempty(ib1)
    ib1 = single(0);
end
if isempty(ic1)
    ic1 = single(0);
end

% 在 Disable = 0 且 Enable = 1 的窗口进行偏置采样
if(Disbale == 0)
    if(Enable == 1)
        ia1 = i1;
        ib1 = i2;
        ic1 = i3;
    end
end

% 偏置赋值
Offset_i1 = ia1;
Offset_i2 = ib1;
Offset_i3 = ic1;

end

== matlab function FOC_Test/Function-Call Subsystem/LPF/LPF ==
  data: input input; output output; Ts input; output_1 input; fc_lpf input
function output = LPF(input, Ts, output_1, fc_lpf)
    

low_pass_factor1 = 2 * pi * fc_lpf * Ts;
low_pass_factor2 = low_pass_factor1 / (1 + low_pass_factor1);

output = low_pass_factor2 * input + (1 - low_pass_factor2) * output_1;

end

== matlab function FOC_Test/Function-Call Subsystem/drive_protect ==
  data: ia input; enable output; ib input; ic input; EN input
function enable = fcn(ia, ib, ic, EN)

persistent en 

if isempty(en)
    en = single(1);
end

% 过流保护
if(EN == 1)
    if ia >= single(5)
        en = single(0);
    elseif ia <= single(-5)
        en = single(0);
    elseif ib >= single(5)
        en = single(0);
    elseif ib <= single(-5)
     en = single(0);
    elseif ic >= single(5)
     en = single(0);
    elseif ic <= single(-5)
        en = single(0);
    end
end

enable = en;
end

== matlab function FOC_Test/Function-Call Subsystem/load_protect ==
  data: speed input; enable output; id input; iq input
function enable = fcn(speed, id, iq)

persistent en 

if isempty(en)
    en = single(1);
end

% 过速保护
if speed >= single(700)
    en = single(0);
elseif speed <= single(-700)
    en = single(0);

% 过流保护
elseif id >= single(5)
    en = single(0);
elseif id <= single(-5)
    en = single(0);
elseif iq >= single(5)
    en = single(0);
elseif iq <= single(-5)
    en = single(0);
end

enable = en;
end

== matlab function FOC_Test/Function-Call Subsystem/offset_get_load ==
  data: Enable input; Offset_i1 output; Disbale input; i1 input; i2 input; i3 input; Offset_i2 output; Offset_i3 output
% 使能时采集电流偏置(采集最近的一次)
function [Offset_i1, Offset_i2, Offset_i3]= offset_get(Enable, Disbale, i1, i2, i3)

% ia1, ib1, ic1 是锁存变量
persistent ia1 ib1 ic1

% 初始化
if isempty(ia1)
    ia1 = single(0);
end
if isempty(ib1)
    ib1 = single(0);
end
if isempty(ic1)
    ic1 = single(0);
end

% 在 Disable = 0 且 Enable = 1 的窗口进行偏置采样
if(Disbale == 0)
    if(Enable == 1)
        ia1 = i1;
        ib1 = i2;
        ic1 = i3;
    end
end

% 偏置赋值
Offset_i1 = ia1;
Offset_i2 = ib1;
Offset_i3 = ic1;

end

== matlab function FOC_Test/Function-Call Subsystem/Clark_load ==
  data: A input; alpha output; B input; C input; beta output
function [alpha, beta] = Clark(A, B, C)

alpha = 2/3 * (A - 0.5 * (B + C));
beta = 2/3 * (sqrt(3)/2 * (B - C));

end

== matlab function FOC_Test/Function-Call Subsystem/Park_load ==
  data: theta input; d output; alpha input; beta input; q output
function [d, q] = Park(theta, alpha, beta)

d = cos(theta) * alpha + sin(theta) * beta;
q = -sin(theta) * alpha + cos(theta) * beta;

end

== matlab function FOC_Test/Function-Call Subsystem/sign ==
  data: speed input; y output
function y = sign(speed)

if speed >= 0
    y = 1;
elseif speed <= -1
    y = -1;
else
    y = 0;
end

== matlab function FOC_Test/Function-Call Subsystem/id_PI_load/PI ==
  data: in input; out output; kp input; ki input; Iout output; EN input; ts input; up input; down input; I input
function [out, Iout] = PI(in, kp, ki, EN, ts, up, down, I)

if(EN == 1)

    % 计算积分输出
    Iout = I + ki * ts * in;

    % 积分限幅
    if(Iout > up)
        Iout = up;
    end
    if(Iout < down)
        Iout = down;
    end
    
    % 合并积分输出和比例输出
    out = kp * in + Iout; 

    % 输出限幅
    if(out > up)
        out = up;
    end
    if(out < down)
        out = down;
    end
else
    Iout = single(0);
    out = single(0);
end
end

== matlab function FOC_Test/Function-Call Subsystem/iq_PI_load/PI ==
  data: in input; out output; kp input; ki input; Iout output; EN input; ts input; up input; down input; I input
function [out, Iout] = PI(in, kp, ki, EN, ts, up, down, I)

if(EN == 1)

    % 计算积分输出
    Iout = I + ki * ts * in;

    % 积分限幅
    if(Iout > up)
        Iout = up;
    end
    if(Iout < down)
        Iout = down;
    end
    
    % 合并积分输出和比例输出
    out = kp * in + Iout; 

    % 输出限幅
    if(out > up)
        out = up;
    end
    if(out < down)
        out = down;
    end
else
    Iout = single(0);
    out = single(0);
end
end
